simulink model "input1"  (R2024b)
settings: Solver=ode4  StartTime=0.0  StopTime=1  FixedStep=1e-4  RelTol=1e-3
undefined symbols (not defined in the file): alphaDeltaVBE, VBE
settings Model: Creator=15054  LastModifiedBy=15054

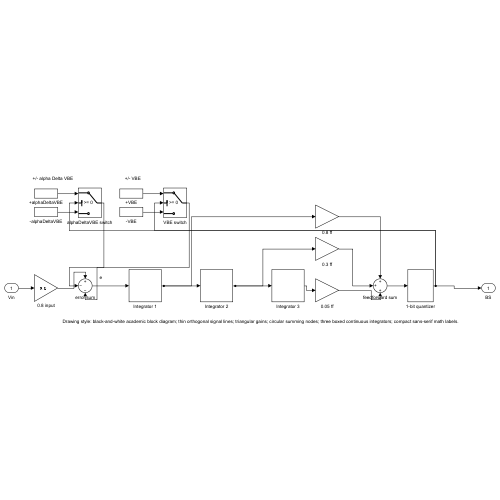
[thumbnail: Simulink's stored preview of the top-level diagram]
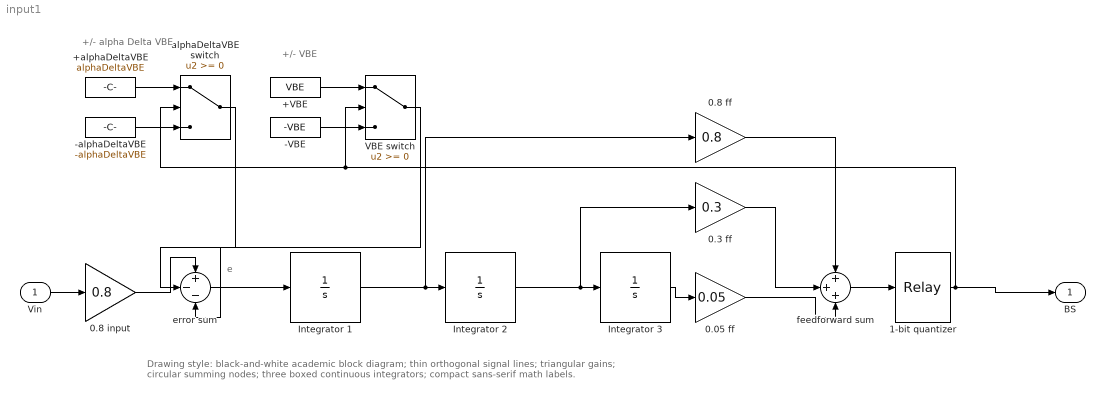
== system input1 ==
  note: Drawing style: black-and-white academic block diagram; thin orthogonal signal lines; triangular gains; circular summing nodes; three boxed continuous integrators; compact sans-serif math labels.
  note: +/- alpha Delta VBE
  note: +/- VBE
  note: e
  Vin : Inport
  +VBE : Constant  Value=VBE
  +alphaDeltaVBE : Constant  Value=alphaDeltaVBE
  -VBE : Constant  Value=-VBE
  -alphaDeltaVBE : Constant  Value=-alphaDeltaVBE
  0.05 ff : Gain  Gain=0.05
  0.3 ff : Gain  Gain=0.3
  0.8 ff : Gain  Gain=0.8
  0.8 input : Gain  Gain=0.8
  1-bit quantizer : Relay  OnSwitchValue=0  OffSwitchValue=0  OffOutputValue=-1
  Integrator 1 : Integrator
  Integrator 2 : Integrator
  Integrator 3 : Integrator
  VBE switch : Switch  SaturateOnIntegerOverflow=off  InputSameDT=off
  alphaDeltaVBE switch : Switch  SaturateOnIntegerOverflow=off  InputSameDT=off
  error sum : Sum  Inputs=+--
  feedforward sum : Sum  Inputs=+++
  BS : Outport
  wires:
  Vin/1 -> 0.8 input/1
  0.8 input/1 -> error sum/1
  error sum/1 -> Integrator 1/1
  Integrator 1/1 -> Integrator 2/1, 0.8 ff/1
  Integrator 2/1 -> Integrator 3/1, 0.3 ff/1
  Integrator 3/1 -> 0.05 ff/1
  0.05 ff/1 -> feedforward sum/3
  feedforward sum/1 -> 1-bit quantizer/1
  1-bit quantizer/1 -> alphaDeltaVBE switch/2, VBE switch/2, BS/1
  0.8 ff/1 -> feedforward sum/1
  0.3 ff/1 -> feedforward sum/2
  +alphaDeltaVBE/1 -> alphaDeltaVBE switch/1
  -alphaDeltaVBE/1 -> alphaDeltaVBE switch/3
  +VBE/1 -> VBE switch/1
  -VBE/1 -> VBE switch/3
  alphaDeltaVBE switch/1 -> error sum/2
  VBE switch/1 -> error sum/3
